simulink model "temperature"  (R2020b)
settings: Solver=VariableStepAuto  StartTime=0.0  StopTime=10.0  RelTol=1e-3
libraries: arduinolib x3
settings Model: Creator=Mostafa Adel  LastModifiedBy=Mostafa Adel

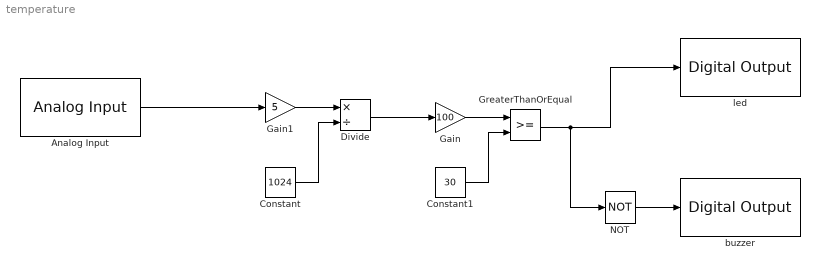
== system temperature ==
  Analog Input : arduinolib/Analog Input  pinNumber=0  ReadResultsOnly=off  ConversionTriggerSource=Software  ExternalTriggerType=uint32( 0 )  OutputDataType=uint16  EnableConversionCompleteNotify=off  EnableOuputStatus=off  SampleTime=-1  blockPlatform=arduino
  Constant : Constant  Value=1024
  Constant1 : Constant  Value=30
  Divide : Product  Inputs=*/
  Gain : Gain  Gain=100
  Gain1 : Gain  Gain=5
  GreaterThanOrEqual : RelationalOperator  OutDataTypeStr=boolean  RndMeth=Simplest
  NOT : Logic  Operator=NOT  IconShape=distinctive  AllPortsSameDT=off  OutDataTypeStr=boolean
  buzzer : arduinolib/Digital Output  pinNumber=9  Direction=output  blockPlatform=arduino
  led : arduinolib/Digital Output  pinNumber=9  Direction=output  blockPlatform=arduino
  wires:
  Analog Input/1 -> Gain1/1
  Gain1/1 -> Divide/1
  Constant/1 -> Divide/2
  Divide/1 -> Gain/1
  Gain/1 -> GreaterThanOrEqual/1
  Constant1/1 -> GreaterThanOrEqual/2
  GreaterThanOrEqual/1 -> NOT/1, led/1
  NOT/1 -> buzzer/1
